simulink model "AUAV3_AND_SLUGS_SENSOR"  (Simulink 7.8)
settings: Solver=FixedStepDiscrete  StartTime=0.0  StopTime=10.0  FixedStep=T  RelTol=1e-3
PreLoadFcn:
  | T = 0.0025;
  | MavlinkBus;
  | 
  | % Baro Altitude Computation
  | % =========================
  | basePressure = 98192.64;
  | baseTemp = 288.215;
  | lapseRate = -0.00198122;
  | baseHeight = 0;
  | 
  | mcuInit
values from neighbouring files (symbols this model uses):
  apSampleTime = 0.01    [mcuInit.m]
  mavlink_gps_raw_int_t = Simulink.Bus    [MavlinkBus.m]    (also in MavlinkBusMarcello.m)
  mavlink_raw_imu_t = Simulink.Bus    [MavlinkBus.m]    (also in MavlinkBusMarcello.m)
  mavlink_scaled_pressure_t = Simulink.Bus    [MavlinkBus.m]    (also in MavlinkBusMarcello.m)
  mavlink_sys_status_t = Simulink.Bus    [MavlinkBus.m]    (also in MavlinkBusMarcello.m)
undefined symbols (not defined in the file or in its folder): A0, A14, A15, A2, A3, A5, A6, B0, barAdjust, baroCutTemp, baroOffset, baroScale, barTGain1, barTGain2, barTMean1, barTMean2, cubeAccelGain16405, cubeGyroGain16405, cubeMagGain16405, D0, D11, D8, G0, G15, gaind, IC1max, lowRateSensorCutoff, mainSensorCutoff, Max, maxDynPressure, ms, OC1max, P112, P127, P16, P21, P30, P31, P64, P72, P75, P80, P82, P83, Pin, pitAdjust, pitCutTemp, pitotOffset, pitotScale, pitTGain1, pitTGain2, pitTMean1, pitTMean2, polesd, powerOffset, powerScale, pressureSensorCutoff, Resol, tempOffset, tempScale ... (+5)
libraries: MCHP_Blockset x56, simulink x21, aerolibconvert2 x2
(part 3 of 5)

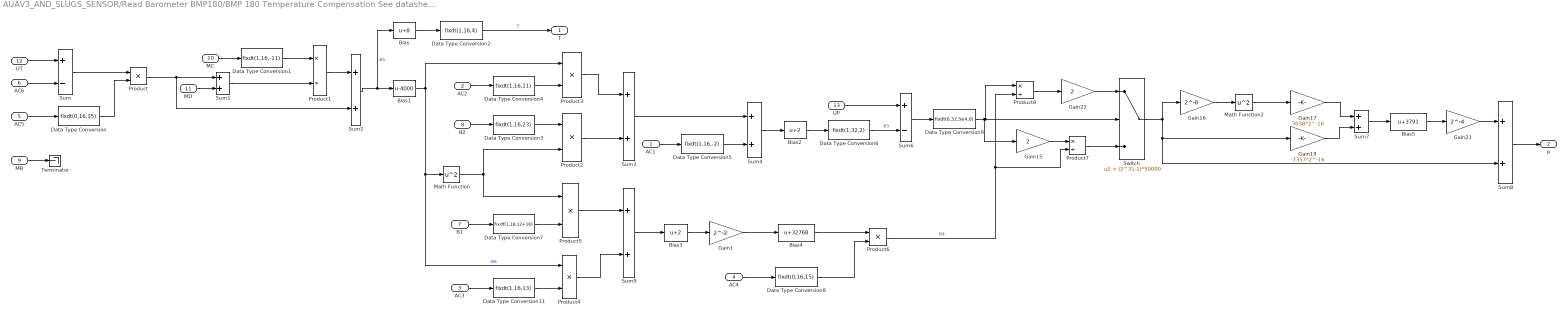
== system AUAV3_AND_SLUGS_SENSOR/Read Barometer BMP180/BMP 180 Temperature Compensation See datasheet ==
  AC1 : Inport
  AC2 : Inport  Port=2
  AC3 : Inport  Port=3
  AC4 : Inport  Port=4
  AC5 : Inport  Port=5
  AC6 : Inport  Port=6
  B1 : Inport  Port=7
  B2 : Inport  Port=8
  MB : Inport  Port=9
  MC : Inport  Port=10
  MD : Inport  Port=11
  UT : Inport  Port=12
  UP : Inport  Port=13
  Bias : Bias  Bias=8
  Bias1 : Bias  Bias=-4000
  Bias2 : Bias  Bias=2
  Bias3 : Bias  Bias=2
  Bias4 : Bias  Bias=32768
  Bias5 : Bias  Bias=3791
  Data Type Conversion : DataTypeConversion  OutDataTypeStr=fixdt(0,16,15)  ConvertRealWorld=Stored Integer (SI)
  Data Type Conversion1 : DataTypeConversion  OutDataTypeStr=fixdt(1,16,-11)  ConvertRealWorld=Stored Integer (SI)
  Data Type Conversion11 : DataTypeConversion  OutDataTypeStr=fixdt(1,16,13)  ConvertRealWorld=Stored Integer (SI)
  Data Type Conversion2 : DataTypeConversion  OutDataTypeStr=fixdt(1,16,4)  ConvertRealWorld=Stored Integer (SI)
  Data Type Conversion3 : DataTypeConversion  OutDataTypeStr=fixdt(1,16,23)  ConvertRealWorld=Stored Integer (SI)
  Data Type Conversion4 : DataTypeConversion  OutDataTypeStr=fixdt(1,16,11)  ConvertRealWorld=Stored Integer (SI)
  Data Type Conversion5 : DataTypeConversion  OutDataTypeStr=fixdt(1,16,-2)  ConvertRealWorld=Stored Integer (SI)
  Data Type Conversion6 : DataTypeConversion  OutDataTypeStr=fixdt(1,32,2)  ConvertRealWorld=Stored Integer (SI)
  Data Type Conversion7 : DataTypeConversion  OutDataTypeStr=fixdt(1,16,12+16)  ConvertRealWorld=Stored Integer (SI)
  Data Type Conversion8 : DataTypeConversion  OutDataTypeStr=fixdt(0,16,15)  ConvertRealWorld=Stored Integer (SI)
  Data Type Conversion9 : DataTypeConversion  OutDataTypeStr=fixdt(0,32,5e4,0)  ConvertRealWorld=Stored Integer (SI)
  Gain1 : Gain  Gain=2^-2  OutDataTypeStr=int32
  Gain15 : Gain  Gain=2  OutDataTypeStr=uint32  RndMeth=Round
  Gain16 : Gain  Gain=2^-8  OutDataTypeStr=int32  RndMeth=Round
  Gain17 : Gain  Gain=3038*2^-16  OutDataTypeStr=uint32
  Gain19 : Gain  Gain=-7357*2^-16  ParamDataTypeStr=fixdt(1,16)  OutDataTypeStr=int32
  Gain21 : Gain  Gain=2^-4  OutDataTypeStr=Inherit: Same as input
  Gain22 : Gain  Gain=2  OutDataTypeStr=Inherit: Same as input
  Math Function : Math  Operator=square  SaturateOnIntegerOverflow=on  OutDataTypeStr=Inherit: Inherit via internal rule
  Math Function2 : Math  Operator=square  OutDataTypeStr=uint32  SaturateOnIntegerOverflow=on
  Product : Product  RndMeth=Round  OutDataTypeStr=Inherit: Same as first input
  Product1 : Product  Inputs=*/  OutDataTypeStr=int16  RndMeth=Round
  Product2 : Product  OutDataTypeStr=int16
  Product3 : Product  OutDataTypeStr=Inherit: Same as first input
  Product4 : Product  OutDataTypeStr=int16
  Product5 : Product  OutDataTypeStr=int16
  Product6 : Product  OutDataTypeStr=uint32
  Product7 : Product  Inputs=*/  RndMeth=Round
  Product8 : Product  Inputs=*/  OutDataTypeStr=uint32  RndMeth=Round
  Sum : Sum  Inputs=+-  RndMeth=Round
  Sum1 : Sum  RndMeth=Round  OutDataTypeStr=Inherit: Same as first input
  Sum2 : Sum  AccumDataTypeStr=int16  OutDataTypeStr=int16  RndMeth=Round
  Sum3 : Sum
  Sum4 : Sum  OutDataTypeStr=int32
  Sum6 : Sum  Inputs=+-  AccumDataTypeStr=uint32  OutDataTypeStr=uint32
  Sum7 : Sum  AccumDataTypeStr=int32  OutDataTypeStr=int32
  Sum8 : Sum  AccumDataTypeStr=int32  OutDataTypeStr=Inherit: Same as accumulator  RndMeth=Round
  Sum9 : Sum
  Switch : Switch  Criteria=u2 > Threshold  Threshold=(2^31-1)*50000
  Terminator : Terminator
  T : Outport
  p : Outport  Port=2
  wires:
  MB/1 -> Terminator/1
  Sum9/1 -> Bias3/1
  Product4/1 -> Sum9/2
  Product5/1 -> Sum9/1
  Product2/1 -> Sum3/2
  Product3/1 -> Sum3/1
  Data Type Conversion3/1 -> Product2/1
  Data Type Conversion11/1 -> Product4/2
  Product1/1 -> Sum2/1
  Data Type Conversion8/1 -> Product6/2
  Data Type Conversion7/1 -> Product5/2
  Data Type Conversion4/1 -> Product3/2
  Math Function/1 -> Product5/1, Product2/2
  Data Type Conversion/1 -> Product/2
  Bias5/1 -> Gain21/1
  Sum8/1 -> p/1
  Gain21/1 -> Sum8/1
  Sum7/1 -> Bias5/1
  Gain17/1 -> Sum7/1
  Gain19/1 -> Sum7/2
  Math Function2/1 -> Gain17/1
  Gain16/1 -> Math Function2/1
  Switch/1 -> Gain19/1, Sum8/2, Gain16/1
  Product7/1 -> Switch/3
  Product8/1 -> Gain22/1
  Data Type Conversion9/1 -> Gain15/1, Product8/1, Switch/2
  Sum6/1 -> Data Type Conversion9/1
  UP/1 -> Sum6/1
  Data Type Conversion6/1 -> Sum6/2  "B3"
  Product6/1 -> Product8/2, Product7/2  "B4"
  Bias4/1 -> Product6/1
  AC4/1 -> Data Type Conversion8/1
  Gain1/1 -> Bias4/1
  Bias3/1 -> Gain1/1
  B1/1 -> Data Type Conversion7/1
  AC3/1 -> Data Type Conversion11/1
  Sum4/1 -> Bias2/1
  Data Type Conversion5/1 -> Sum4/2
  Bias2/1 -> Data Type Conversion6/1
  AC1/1 -> Data Type Conversion5/1
  Sum3/1 -> Sum4/1
  AC2/1 -> Data Type Conversion4/1
  B2/1 -> Data Type Conversion3/1
  Bias1/1 -> Product3/1, Product4/1, Math Function/1  "B6"
  MC/1 -> Data Type Conversion1/1
  Data Type Conversion2/1 -> T/1  "T"
  Bias/1 -> Data Type Conversion2/1
  Sum1/1 -> Product1/2
  Sum2/1 -> Bias1/1, Bias/1  "B5"
  Product/1 -> Sum1/1, Sum2/2
  MD/1 -> Sum1/2
  AC5/1 -> Data Type Conversion/1
  Sum/1 -> Product/1
  AC6/1 -> Sum/2
  UT/1 -> Sum/1
  Data Type Conversion1/1 -> Product1/1
  Gain22/1 -> Switch/1
  Gain15/1 -> Product7/1

== system AUAV3_AND_SLUGS_SENSOR/Read Barometer BMP180/Baro Altimeter ==
  Static (Pa) : Inport
  Compute Barometric Height : Subsystem  mask{baseTemp=baseTemp, LapseRate=lapseRate}
      mask prompts: baseTemp "Base Station Temperature (K)"; LapseRate "Lapse Rate (C/ft)"
      mask help:
      | Produces Altitude in meters from Barometric Pressure in Pascals. Altitude is valid from MSL to 6000 ft.
      |
      | The method implemented here was developed by Ren Curry
  Constant5 : Constant  Value=baseHeight  OutDataTypeStr=single
  Enabled Subsystem : Subsystem  TreatAsAtomicUnit=on
  Enables/Disables the Computation of  initial Baro Bias : MATLAB Function  TreatAsAtomicUnit=on
  Initial Baro Bias : Subsystem  TreatAsAtomicUnit=on
  Logical Operator : Logic  Operator=NOT  AllPortsSameDT=off  OutDataTypeStr=boolean
  Sum1 : Sum  Inputs=++|  OutDataTypeStr=single
  Zero Out Height : Subsystem  TreatAsAtomicUnit=on
  Altitude : Outport
  wires:
  Enabled Subsystem/1(Out1) -> Altitude/1
  Sum1/1 -> Enabled Subsystem/1(In1)
  Logical Operator/1 -> Enabled Subsystem/Enable
  Zero Out Height/1(Height Offset) -> Sum1/1
  Initial Baro Bias/1(Baro (Gnd)) -> Compute Barometric Height/2(Base Pressure (Pa))
  Constant5/1 -> Zero Out Height/1(Base Height), Compute Barometric Height/1(Base Height (m))
  Enables/Disables the Computation of  initial Baro Bias/1(tOut) -> Logical Operator/1, Zero Out Height/Enable, Initial Baro Bias/Enable
  Static (Pa)/1 -> Compute Barometric Height/3(Baro (Pa)), Initial Baro Bias/1(Baro (Pa))
  Compute Barometric Height/1("Altitude, m") -> Sum1/2, Zero Out Height/2(Computed Height)

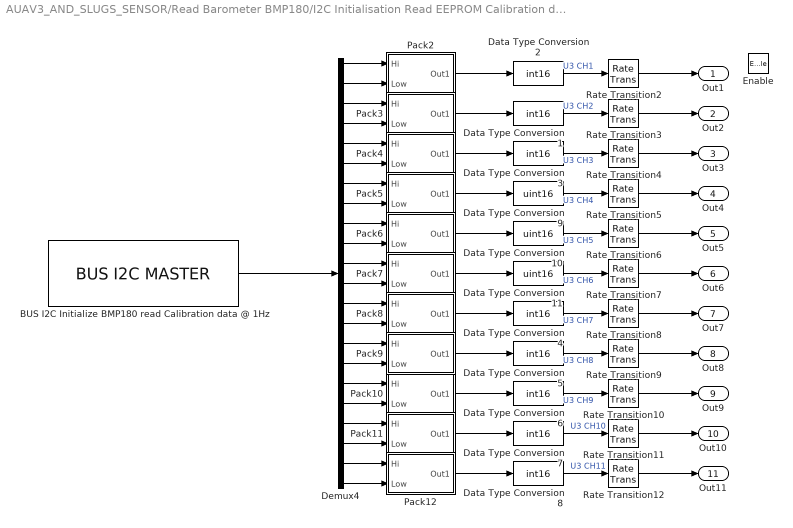
== system AUAV3_AND_SLUGS_SENSOR/Read Barometer BMP180/I2C Initialisation Read EEPROM Calibration data Once (Blocking Function) ==
  Enable : EnablePort
  BUS I2C Initialize BMP180 read Calibration data @ 1Hz : MCHP_Blockset/BUS I2C/BUS I2C MASTER  I2CRef=2  I2C_IntPriority=6  I2Csequence_txt="Initial-Configuration$     ---     $Start$Write Address:{[0x77]}    % BMP180 Address$Write Data (x1)  Write:{[0xAA ]}  $Re-Start    % Re-Start when not followed with either Read or Write action rethrow Address$Read Data (x22)  Read:{Out 9}$Stop"  I2Csequence_num=[BFF0000000000000 40E0600000000000 41186A0000000000 4118666E3C87173F]$[4070000000000000]$[3FF0000000000000 40E0200000000000 40F86A0000000000 40F866E066594CA2]$[4040000000000000 0000000000000000 0000000000000000 405DC00000000000]$[4050000000000000 3FF0000000000000 0000000000000000 4065400000000000]$[4008000000000000 40E0000000000000 40F86A0000000000 410065D9C7810E65]$[4060000000000000 4036000000000000]$[4000000000000000 40E0600000000000 40F86A0000000000 410065D9C7810E65]  InitialConfigurationNum=0  PIN_SDA_TXT=A3 / Pin[59]  PIN_SCL_TXT=A2 / Pin[58]  S_INPUT="[5  5]"  S_OUTPUT=[5]  S_INPUT_Size="[2  2]"  S_OUTPUT_Size=[4]  BlockingMode=on  SampleTime=.01  MCHP_MASTERLINK=|  MCHP_PORT={I2C 2 Clock}{SCL2}13:0:A2;{I2C 2 SDA}{SDA2}13:0:A3;  ORDERING=0
      | AUAV3_AND_SLUGS_SENSOR/Microchip Master
      | AUAV V3 Board
      | Busy Flag on D2 (RA6)
  Data Type Conversion{1..8} (8 alike) : DataTypeConversion  OutDataTypeStr=int16  ConvertRealWorld=Stored Integer (SI)
  Data Type Conversion10 : DataTypeConversion  OutDataTypeStr=uint16  ConvertRealWorld=Stored Integer (SI)  LockScale=on
  Data Type Conversion11 : DataTypeConversion  OutDataTypeStr=uint16  ConvertRealWorld=Stored Integer (SI)  LockScale=on
  Data Type Conversion9 : DataTypeConversion  OutDataTypeStr=uint16  ConvertRealWorld=Stored Integer (SI)  LockScale=on
  Demux4 : Demux  Outputs=22
  Pack10 : Subsystem
  Pack11 : Subsystem
  Pack12 : Subsystem
  Pack2 : Subsystem
  Pack3 : Subsystem
  Pack4 : Subsystem
  Pack5 : Subsystem
  Pack6 : Subsystem
  Pack7 : Subsystem
  Pack8 : Subsystem
  Pack9 : Subsystem
  Rate Transition{2..12} (11 alike) : RateTransition  Deterministic=off
  Out1 : Outport
  Out2 : Outport  Port=2
  Out3 : Outport  Port=3
  Out4 : Outport  Port=4
  Out5 : Outport  Port=5
  Out6 : Outport  Port=6
  Out7 : Outport  Port=7
  Out8 : Outport  Port=8
  Out9 : Outport  Port=9
  Out10 : Outport  Port=10
  Out11 : Outport  Port=11
  wires:
  BUS I2C Initialize BMP180 read Calibration data @ 1Hz/1 -> Demux4/1
  Demux4/12 -> Pack7/2(Low)
  Data Type Conversion10/1 -> Rate Transition6/1  "U3 CH5"
  Data Type Conversion1/1 -> Rate Transition3/1  "U3 CH2"
  Data Type Conversion2/1 -> Rate Transition2/1  "U3 CH1"
  Data Type Conversion11/1 -> Rate Transition7/1  "U3 CH6"
  Data Type Conversion5/1 -> Rate Transition9/1  "U3 CH8"
  Data Type Conversion8/1 -> Rate Transition12/1  "U3 CH11"
  Data Type Conversion6/1 -> Rate Transition10/1  "U3 CH9"
  Data Type Conversion4/1 -> Rate Transition8/1  "U3 CH7"
  Data Type Conversion3/1 -> Rate Transition4/1  "U3 CH3"
  Data Type Conversion7/1 -> Rate Transition11/1  "U3 CH10"
  Data Type Conversion9/1 -> Rate Transition5/1  "U3 CH4"
  Pack6/1(Out1) -> Data Type Conversion10/1
  Pack5/1(Out1) -> Data Type Conversion9/1
  Pack7/1(Out1) -> Data Type Conversion11/1
  Pack8/1(Out1) -> Data Type Conversion4/1
  Pack9/1(Out1) -> Data Type Conversion5/1
  Pack10/1(Out1) -> Data Type Conversion6/1
  Pack11/1(Out1) -> Data Type Conversion7/1
  Pack12/1(Out1) -> Data Type Conversion8/1
  Pack4/1(Out1) -> Data Type Conversion3/1
  Demux4/15 -> Pack9/1(Hi)
  Pack3/1(Out1) -> Data Type Conversion1/1
  Pack2/1(Out1) -> Data Type Conversion2/1
  Demux4/22 -> Pack12/2(Low)
  Demux4/14 -> Pack8/2(Low)
  Demux4/16 -> Pack9/2(Low)
  Demux4/17 -> Pack10/1(Hi)
  Demux4/18 -> Pack10/2(Low)
  Demux4/19 -> Pack11/1(Hi)
  Demux4/20 -> Pack11/2(Low)
  Demux4/21 -> Pack12/1(Hi)
  Demux4/2 -> Pack2/2(Low)
  Demux4/13 -> Pack8/1(Hi)
  Demux4/11 -> Pack7/1(Hi)
  Demux4/9 -> Pack6/1(Hi)
  Demux4/10 -> Pack6/2(Low)
  Demux4/1 -> Pack2/1(Hi)
  Demux4/3 -> Pack3/1(Hi)
  Demux4/4 -> Pack3/2(Low)
  Demux4/6 -> Pack4/2(Low)
  Demux4/5 -> Pack4/1(Hi)
  Demux4/7 -> Pack5/1(Hi)
  Demux4/8 -> Pack5/2(Low)
  Rate Transition12/1 -> Out11/1
  Rate Transition10/1 -> Out9/1
  Rate Transition11/1 -> Out10/1
  Rate Transition9/1 -> Out8/1
  Rate Transition3/1 -> Out2/1
  Rate Transition7/1 -> Out6/1
  Rate Transition4/1 -> Out3/1
  Rate Transition6/1 -> Out5/1
  Rate Transition8/1 -> Out7/1
  Rate Transition2/1 -> Out1/1
  Rate Transition5/1 -> Out4/1

== system AUAV3_AND_SLUGS_SENSOR/Read Barometer BMP180/LPF 1Hz ==
  Input : Inport
  Delay11 : Delay  DelayLength=1  InitialCondition=0  InputProcessing=Inherited
  SumA21 : Sum  Inputs=|++  AccumDataTypeStr=fixdt(0,32,15)  OutDataTypeStr=Inherit: Same as accumulator  SaturateOnIntegerOverflow=on
  SumB21 : Sum  Inputs=|++  AccumDataTypeStr=fixdt(0,32,16)  OutDataTypeStr=uint16  SaturateOnIntegerOverflow=on
  a(2)(1) : Gain  Gain=0.9390625058174924  ParamDataTypeStr=fixdt(0,16,16)  OutDataTypeStr=fixdt(0,32,15)  SaturateOnIntegerOverflow=on
  s(1) : Gain  Gain=0.030468747091253828  ParamDataTypeStr=fixdt(0,16,20)  OutDataTypeStr=fixdt(0,32,16)  SaturateOnIntegerOverflow=on
  Output : Outport
  wires:
  s(1)/1 -> SumA21/1
  SumA21/1 -> SumB21/1, Delay11/1
  a(2)(1)/1 -> SumA21/2
  Delay11/1 -> SumB21/2, a(2)(1)/1
  SumB21/1 -> Output/1
  Input/1 -> s(1)/1

== system AUAV3_AND_SLUGS_SENSOR/Read Barometer BMP180/LPF 1Hz1 ==
  Input : Inport
  Delay11 : Delay  DelayLength=1  InitialCondition=0  InputProcessing=Inherited
  SumA21 : Sum  Inputs=|++  AccumDataTypeStr=fixdt(0,32,15)  OutDataTypeStr=Inherit: Same as accumulator  SaturateOnIntegerOverflow=on
  SumB21 : Sum  Inputs=|++  AccumDataTypeStr=fixdt(0,32,16)  OutDataTypeStr=uint16  SaturateOnIntegerOverflow=on
  a(2)(1) : Gain  Gain=0.9390625058174924  ParamDataTypeStr=fixdt(0,16,16)  OutDataTypeStr=fixdt(0,32,15)  SaturateOnIntegerOverflow=on
  s(1) : Gain  Gain=0.030468747091253828  ParamDataTypeStr=fixdt(0,16,20)  OutDataTypeStr=fixdt(0,32,16)  SaturateOnIntegerOverflow=on
  Output : Outport
  wires:
  Input/1 -> s(1)/1
  SumB21/1 -> Output/1
  Delay11/1 -> a(2)(1)/1, SumB21/2
  a(2)(1)/1 -> SumA21/2
  SumA21/1 -> Delay11/1, SumB21/1
  s(1)/1 -> SumA21/1

== system AUAV3_AND_SLUGS_SENSOR/Read Barometer BMP180/Pack ==
  Hi : Inport
  Low : Inport  Port=2
  Bitwise Operator : simulink/Logic and Bit Operations/Bitwise Operator  logicop=OR  UseBitMask=off  NumInputPorts=2  BitMask=bin2dec('11011001')  BitMaskRealWorld=Stored Integer
  Data Type Conversion1 : DataTypeConversion  OutDataTypeStr=uint16  ConvertRealWorld=Stored Integer (SI)
  Data Type Conversion2 : DataTypeConversion  OutDataTypeStr=uint16  ConvertRealWorld=Stored Integer (SI)
  Data Type Conversion3 : DataTypeConversion  OutDataTypeStr=uint16  ConvertRealWorld=Stored Integer (SI)
  Gain : Gain  Gain=2^8  OutDataTypeStr=Inherit: Same as input
  Out1 : Outport
  wires:
  Data Type Conversion3/1 -> Bitwise Operator/2
  Low/1 -> Data Type Conversion3/1
  Data Type Conversion1/1 -> Gain/1
  Bitwise Operator/1 -> Data Type Conversion2/1
  Hi/1 -> Data Type Conversion1/1
  Gain/1 -> Bitwise Operator/1
  Data Type Conversion2/1 -> Out1/1

== system AUAV3_AND_SLUGS_SENSOR/Read Barometer BMP180/Pack1 ==
  Hi : Inport
  Low : Inport  Port=2
  Bitwise Operator : simulink/Logic and Bit Operations/Bitwise Operator  logicop=OR  UseBitMask=off  NumInputPorts=2  BitMask=bin2dec('11011001')  BitMaskRealWorld=Stored Integer
  Data Type Conversion1 : DataTypeConversion  OutDataTypeStr=uint16  ConvertRealWorld=Stored Integer (SI)
  Data Type Conversion2 : DataTypeConversion  OutDataTypeStr=uint16  ConvertRealWorld=Stored Integer (SI)
  Data Type Conversion3 : DataTypeConversion  OutDataTypeStr=uint16  ConvertRealWorld=Stored Integer (SI)
  Gain : Gain  Gain=2^8  OutDataTypeStr=Inherit: Same as input
  Out1 : Outport
  wires:
  Gain/1 -> Bitwise Operator/1
  Hi/1 -> Data Type Conversion1/1
  Bitwise Operator/1 -> Data Type Conversion2/1
  Data Type Conversion1/1 -> Gain/1
  Low/1 -> Data Type Conversion3/1
  Data Type Conversion3/1 -> Bitwise Operator/2
  Data Type Conversion2/1 -> Out1/1

== system AUAV3_AND_SLUGS_SENSOR/Read MPU600 and HMC5883/Subsystem10 ==
  Hi : Inport
  Low : Inport  Port=2
  Bitwise Operator : simulink/Logic and Bit Operations/Bitwise Operator  logicop=OR  UseBitMask=off  NumInputPorts=2  BitMask=bin2dec('11011001')  BitMaskRealWorld=Stored Integer
  Data Type Conversion1 : DataTypeConversion  OutDataTypeStr=uint16  ConvertRealWorld=Stored Integer (SI)
  Data Type Conversion2 : DataTypeConversion  OutDataTypeStr=int16  ConvertRealWorld=Stored Integer (SI)
  Data Type Conversion3 : DataTypeConversion  OutDataTypeStr=uint16  ConvertRealWorld=Stored Integer (SI)
  Shift Arithmetic : ArithShift  BitShiftNumber=8
  Out1 : Outport
  wires:
  Hi/1 -> Data Type Conversion1/1
  Bitwise Operator/1 -> Data Type Conversion2/1
  Data Type Conversion2/1 -> Out1/1
  Data Type Conversion1/1 -> Shift Arithmetic/1
  Shift Arithmetic/1 -> Bitwise Operator/1
  Low/1 -> Data Type Conversion3/1
  Data Type Conversion3/1 -> Bitwise Operator/2

== system AUAV3_AND_SLUGS_SENSOR/Read MPU600 and HMC5883/Subsystem8 ==
  Hi : Inport
  Low : Inport  Port=2
  Bitwise Operator : simulink/Logic and Bit Operations/Bitwise Operator  logicop=OR  UseBitMask=off  NumInputPorts=2  BitMask=bin2dec('11011001')  BitMaskRealWorld=Stored Integer
  Data Type Conversion1 : DataTypeConversion  OutDataTypeStr=uint16  ConvertRealWorld=Stored Integer (SI)
  Data Type Conversion2 : DataTypeConversion  OutDataTypeStr=int16  ConvertRealWorld=Stored Integer (SI)
  Data Type Conversion3 : DataTypeConversion  OutDataTypeStr=uint16  ConvertRealWorld=Stored Integer (SI)
  Shift Arithmetic : ArithShift  BitShiftNumber=8
  Out1 : Outport
  wires:
  Hi/1 -> Data Type Conversion1/1
  Bitwise Operator/1 -> Data Type Conversion2/1
  Data Type Conversion2/1 -> Out1/1
  Data Type Conversion1/1 -> Shift Arithmetic/1
  Shift Arithmetic/1 -> Bitwise Operator/1
  Low/1 -> Data Type Conversion3/1
  Data Type Conversion3/1 -> Bitwise Operator/2

== system AUAV3_AND_SLUGS_SENSOR/Read MPU600 and HMC5883/Subsystem9 ==
  Hi : Inport
  Low : Inport  Port=2
  Bitwise Operator : simulink/Logic and Bit Operations/Bitwise Operator  logicop=OR  UseBitMask=off  NumInputPorts=2  BitMask=bin2dec('11011001')  BitMaskRealWorld=Stored Integer
  Data Type Conversion1 : DataTypeConversion  OutDataTypeStr=uint16  ConvertRealWorld=Stored Integer (SI)
  Data Type Conversion2 : DataTypeConversion  OutDataTypeStr=int16  ConvertRealWorld=Stored Integer (SI)
  Data Type Conversion3 : DataTypeConversion  OutDataTypeStr=uint16  ConvertRealWorld=Stored Integer (SI)
  Shift Arithmetic : ArithShift  BitShiftNumber=8
  Out1 : Outport
  wires:
  Data Type Conversion3/1 -> Bitwise Operator/2
  Low/1 -> Data Type Conversion3/1
  Shift Arithmetic/1 -> Bitwise Operator/1
  Data Type Conversion1/1 -> Shift Arithmetic/1
  Data Type Conversion2/1 -> Out1/1
  Bitwise Operator/1 -> Data Type Conversion2/1
  Hi/1 -> Data Type Conversion1/1

== system AUAV3_AND_SLUGS_SENSOR/Sensor Data/Raw HIL  Readings ==
  Enable : EnablePort
  Data from HIL [hil.c]2 : MCHP_Blockset/User Functions/C Function Call  ParseFilesChkbx=off  ListFunctions1=Custom Function  Function1=extern void hilRead(uint8_T* y1);  AddHeaderDeclaration=off  Function1Type=when block is updated (default)  FctReturnBlockOut=on  Fct1BlockOut=y1[13]  DataCollected=0  ORDERING=None  SampleTime=.01  MCHP_MASTERLINK=|  PinDigitalInput=[]  PinDigitalOutput=[]  PinAnalogInput=[]
      | AUAV3_AND_SLUGS_SENSOR/Microchip Master
      | AUAV V3 Board
      | Busy Flag on D2 (RA6)
  HIL Messages  Parser/Decoder [hil.c]1 : MCHP_Blockset/User Functions/C Function Call  ParseFilesChkbx=off  ListFunctions1=Custom Function  Function1=extern void protDecodeHil(uint8_T* u1);  AddHeaderDeclaration=off  Function1Type=when block is updated (default)  Fct1BlockIn=u1[13]  FctReturnBlockOut=off  Fct1BlockOut=u1[13]  DataCollected=0  ORDERING=None  SampleTime=-1  MCHP_MASTERLINK=|  PinDigitalInput=[]  PinDigitalOutput=[]  PinAnalogInput=[]
      | AUAV3_AND_SLUGS_SENSOR/Microchip Master
      | AUAV V3 Board
      | Busy Flag on D2 (RA6)
  HIL Raw Readings [hil.c]1 : MCHP_Blockset/User Functions/C Function Call  ParseFilesChkbx=off  ListFunctions1=Custom Function  Function1=extern void hil_getRawRead(uint8_T* y1);  AddHeaderDeclaration=off  Function1Type=when block is updated (default)  Fct1BlockIn=y1[13]  FctReturnBlockOut=off  Fct1BlockOut=y1[13]  ORDERING=None  SampleTime=-1  MCHP_MASTERLINK=|  PinDigitalInput=[]  PinDigitalOutput=[]  PinAnalogInput=[]
      | AUAV3_AND_SLUGS_SENSOR/Microchip Master
      | AUAV V3 Board
      | Busy Flag on D2 (RA6)
  Raw Msg : Outport
  wires:
  Data from HIL [hil.c]2/1 -> HIL Messages  Parser/Decoder [hil.c]1/1
  HIL Messages  Parser/Decoder [hil.c]1/1 -> HIL Raw Readings [hil.c]1/1
  HIL Raw Readings [hil.c]1/1 -> Raw Msg/1

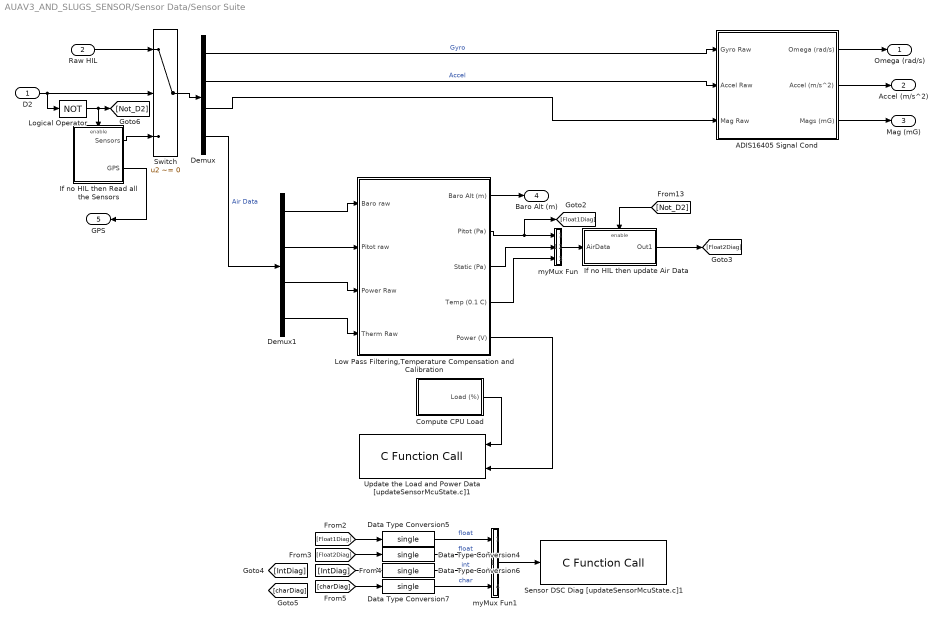
== system AUAV3_AND_SLUGS_SENSOR/Sensor Data/Sensor Suite ==
  D2 : Inport
  Raw HIL : Inport  Port=2
  "ADIS16405 Signal Cond " : Subsystem
  Compute CPU Load : Subsystem
  Data Type Conversion{4..7} (4 alike) : DataTypeConversion  OutDataTypeStr=single
  Demux : Demux  Outputs=[3 3 3 4]
  Demux1 : Demux
  If no HIL then Read all the Sensors : Subsystem
  If no HIL then update Air Data : Subsystem
  Logical Operator : Logic  Operator=NOT  AllPortsSameDT=off  OutDataTypeStr=boolean
  Low Pass Filtering,Temperature Compensation and Calibration : Subsystem
  Sensor DSC Diag [updateSensorMcuState.c]1 : MCHP_Blockset/User Functions/C Function Call  ParseFilesChkbx=off  ListFunctions1=Custom Function  Function1=extern void updateSensorDiag(real32_T* u1);  AddHeaderDeclaration=off  Function1Type=when block is updated (default)  Fct1BlockIn=u1[4]  FctReturnBlockOut=off  DataCollected=0  ORDERING=None  SampleTime=.01  MCHP_MASTERLINK=|  PinDigitalInput=[]  PinDigitalOutput=[]  PinAnalogInput=[]
      | AUAV3_AND_SLUGS_SENSOR/Microchip Master
      | AUAV V3 Board
      | Busy Flag on D2 (RA6)
  Switch : Switch  Criteria=u2 ~= 0  SampleTime=0.01
  Update the Load and Power Data [updateSensorMcuState.c]1 : MCHP_Blockset/User Functions/C Function Call  ParseFilesChkbx=off  ListFunctions1=Custom Function  Function1=extern void updateLoadData(uint8_T u1, uint16_T u2);  AddHeaderDeclaration=off  Function1Type=when block is updated (default)  FctReturnBlockOut=off  DataCollected=0  ORDERING=None  SampleTime=.01  MCHP_MASTERLINK=|  PinDigitalInput=[]  PinDigitalOutput=[]  PinAnalogInput=[]
      | AUAV3_AND_SLUGS_SENSOR/Microchip Master
      | AUAV V3 Board
      | Busy Flag on D2 (RA6)
  myMux Fun : MATLAB Function  TreatAsAtomicUnit=on
  myMux Fun1 : MATLAB Function  TreatAsAtomicUnit=on
  Omega (rad/s) : Outport
  Accel (m/s^2) : Outport  Port=2
  Mag (mG) : Outport  Port=3
  Baro Alt (m) : Outport  Port=4
  GPS : Outport  Port=5
  wires:
  Switch/1 -> Demux/1
  D2/1 -> Switch/2, Logical Operator/1
  If no HIL then Read all the Sensors/1(Sensors) -> Switch/3
  Logical Operator/1 -> If no HIL then Read all the Sensors/Enable, [Not_D2]
  Raw HIL/1 -> Switch/1
  Low Pass Filtering,Temperature Compensation and Calibration/1(Baro Alt (m)) -> Baro Alt (m)/1
  Demux/1 -> "ADIS16405 Signal Cond "/1(Gyro Raw)  "Gyro"
  Demux/4 -> Demux1/1  "Air Data"
  Demux1/1 -> Low Pass Filtering,Temperature Compensation and Calibration/1(Baro raw)
  Demux1/2 -> Low Pass Filtering,Temperature Compensation and Calibration/2(Pitot raw)
  Demux1/4 -> Low Pass Filtering,Temperature Compensation and Calibration/4(Therm Raw)
  Demux/3 -> "ADIS16405 Signal Cond "/3(Mag Raw)
  Demux1/3 -> Low Pass Filtering,Temperature Compensation and Calibration/3(Power Raw)
  Low Pass Filtering,Temperature Compensation and Calibration/2(Pitot (Pa)) -> myMux Fun/1(u1), [Float1Diag]
  Low Pass Filtering,Temperature Compensation and Calibration/3(Static (Pa)) -> myMux Fun/2(u2)
  myMux Fun/1(y) -> If no HIL then update Air Data/1(AirData)
  Low Pass Filtering,Temperature Compensation and Calibration/4(Temp (0.1 C)) -> myMux Fun/3(u3)
  Compute CPU Load/1(Load (%)) -> Update the Load and Power Data [updateSensorMcuState.c]1/1
  Low Pass Filtering,Temperature Compensation and Calibration/5(Power (V)) -> Update the Load and Power Data [updateSensorMcuState.c]1/2
  If no HIL then Read all the Sensors/2(GPS) -> GPS/1
  Demux/2 -> "ADIS16405 Signal Cond "/2(Accel Raw)  "Accel"
  myMux Fun1/1(y) -> Sensor DSC Diag [updateSensorMcuState.c]1/1
  Data Type Conversion5/1 -> myMux Fun1/1(u1)  "float"
  Data Type Conversion4/1 -> myMux Fun1/2(u2)  "float"
  Data Type Conversion6/1 -> myMux Fun1/3(u3)  "int"
  Data Type Conversion7/1 -> myMux Fun1/4(u4)  "char"
  [Float1Diag] -> Data Type Conversion5/1
  [Float2Diag] -> Data Type Conversion4/1
  [IntDiag] -> Data Type Conversion6/1
  [charDiag] -> Data Type Conversion7/1
  "ADIS16405 Signal Cond "/1(Omega (rad/s)) -> Omega (rad/s)/1
  "ADIS16405 Signal Cond "/2(Accel (m/s^2)) -> Accel (m/s^2)/1
  "ADIS16405 Signal Cond "/3(Mags (mG)) -> Mag (mG)/1
  [Not_D2] -> If no HIL then update Air Data/Enable
  If no HIL then update Air Data/1(Out1) -> [Float2Diag]

== system AUAV3_AND_SLUGS_SENSOR/Servo In Out/Mixing ==
  note: Pitch positif : go down
      | Yaw positive : turn left
  Pitch : Inport
  Roll : Inport  Port=2
  Sum : Sum  Inputs=-+  SaturateOnIntegerOverflow=on  OutDataTypeStr=Inherit: Same as first input
  Sum1 : Sum  SaturateOnIntegerOverflow=on  OutDataTypeStr=Inherit: Same as first input
  Cmd Servo Left : Outport
  Cmd Servo Right : Outport  Port=2
  wires:
  Pitch/1 -> Sum1/1, Sum/1
  Roll/1 -> Sum/2, Sum1/2
  Sum/1 -> Cmd Servo Left/1
  Sum1/1 -> Cmd Servo Right/1

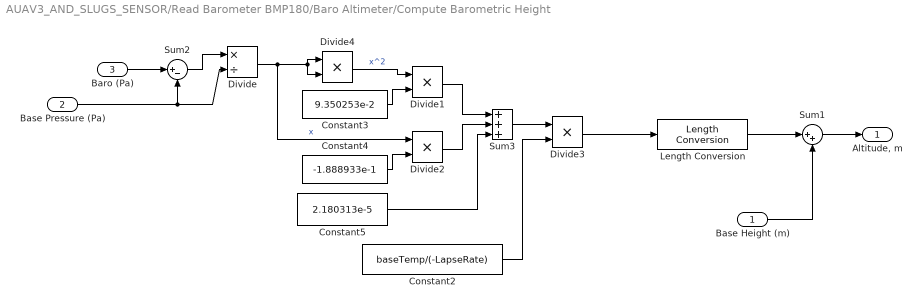
== system AUAV3_AND_SLUGS_SENSOR/Read Barometer BMP180/Baro Altimeter/Compute Barometric Height ==
  Base Height (m) : Inport
  Base Pressure (Pa) : Inport  Port=2
  Baro (Pa) : Inport  Port=3
  Constant2 : Constant  Value=baseTemp/(-LapseRate)  OutDataTypeStr=single
  Constant3 : Constant  Value=9.350253e-2  OutDataTypeStr=single
  Constant4 : Constant  Value=-1.888933e-1  OutDataTypeStr=single
  Constant5 : Constant  Value=2.180313e-5  OutDataTypeStr=single
  Divide : Product  Inputs=*/  OutDataTypeStr=single
  Divide{1..4} (4 alike) : Product  OutDataTypeStr=single
  Length Conversion : aerolibconvert2/Length Conversion  IU=ft  OU=m
  Sum1 : Sum  Inputs=|++  OutDataTypeStr=single
  Sum2 : Sum  Inputs=|+-  OutDataTypeStr=single
  Sum3 : Sum  Inputs=3  OutDataTypeStr=single
  "Altitude, m" : Outport
  wires:
  Baro (Pa)/1 -> Sum2/1
  Base Height (m)/1 -> Sum1/2
  Base Pressure (Pa)/1 -> Sum2/2, Divide/2
  Divide/1 -> Divide4/2, Divide4/1, Divide2/1  "x"
  Divide4/1 -> Divide1/1  "x^2"
  Constant3/1 -> Divide1/2
  Constant4/1 -> Divide2/2
  Divide1/1 -> Sum3/1
  Divide2/1 -> Sum3/2
  Constant5/1 -> Sum3/3
  Sum3/1 -> Divide3/1
  Constant2/1 -> Divide3/2
  Divide3/1 -> Length Conversion/1
  Sum1/1 -> "Altitude, m"/1
  Sum2/1 -> Divide/1
  Length Conversion/1 -> Sum1/1

== system AUAV3_AND_SLUGS_SENSOR/Read Barometer BMP180/Baro Altimeter/Enabled Subsystem ==
  In1 : Inport
  Enable : EnablePort
  Out1 : Outport  InitialOutput=baseHeight
  wires:
  In1/1 -> Out1/1

== system AUAV3_AND_SLUGS_SENSOR/Read Barometer BMP180/Baro Altimeter/Initial Baro Bias ==
  Baro (Pa) : Inport
  Enable : EnablePort
  Data Type Conversion : DataTypeConversion  OutDataTypeStr=double
  Data Type Conversion1 : DataTypeConversion  OutDataTypeStr=single
  Low Pass8 : Subsystem  mask(DiscretizedZeroPole){Zeros=[], Poles=[-3], Gain=3, AbsTol=auto, SampleTime=.01, method=tustin, Wc=1}
      mask prompts: Zeros "Zeros (enter in s-main:)"; Poles "Poles (enter in s-domain:)"; Gain "Gain (enter in s-domain:)"; AbsTol "Absolute tolerance:"; SampleTime "Sample time:"; Wc "Critical Frequency (Hz):"
      mask help: Continuous mask uses c2d to transform parameters onto the Discrete Zero-Pole block inside.
      mask init:
      | st=SampleTime;
      | if length(st)>1
      |     st=SampleTime(1);
      | end
      | if(st>0)
      |     [zerosd,polesd,gaind] = sldiscutil('disczpk', {st,method,Wc,Zeros,Poles,Gain});
      | end	
      | s = get_param(gcb,'maskvalues');
      | zeross = s{1};
      | poless = s{2};
      | gainss = s{3};
      | %zerosc = eval(zeross);
      | %polesc = eval(poless);
      | %gainsc = eval(gainss);
      | sldiscutil('initzpkmask', st);
      | if(st==0)
      | set_param([gcb '/Zero Pole'], 'AbsoluteTolerance', AbsTol);
      | end
      mask StyleString: edit,edit,edit,edit,edit,popup(zoh|foh|tustin|prewarp|matched),edit
      mask CallbackString: |||||hidecrit|
      mask Display:
      | droots(zeross,poless,gainss)
      | text( 0.5, 1.0, method, 'verticalAlignment','top')
  "[80k - 120k]" : Saturate  UpperLimit=120000  LowerLimit=80000
  Baro (Gnd) : Outport
  wires:
  "[80k - 120k]"/1 -> Baro (Gnd)/1
  Data Type Conversion1/1 -> "[80k - 120k]"/1
  Data Type Conversion/1 -> Low Pass8/1(In1)
  Low Pass8/1(Out1) -> Data Type Conversion1/1
  Baro (Pa)/1 -> Data Type Conversion/1

== system AUAV3_AND_SLUGS_SENSOR/Read Barometer BMP180/Baro Altimeter/Zero Out Height ==
  Base Height : Inport
  Computed Height : Inport  Port=2
  Enable : EnablePort
  Integer Delay : Delay  DelayLength=1  InitialCondition=0  InputProcessing=Inherited  SampleTime=.01
  Sum : Sum  Inputs=|+-  OutDataTypeStr=single
  Height Offset : Outport
  wires:
  Base Height/1 -> Sum/1
  Integer Delay/1 -> Sum/2
  Sum/1 -> Height Offset/1
  Computed Height/1 -> Integer Delay/1

== system AUAV3_AND_SLUGS_SENSOR/Read Barometer BMP180/I2C Initialisation Read EEPROM Calibration data Once (Blocking Function)/Pack10 ==
  Hi : Inport
  Low : Inport  Port=2
  Bitwise Operator : simulink/Logic and Bit Operations/Bitwise Operator  logicop=OR  UseBitMask=off  NumInputPorts=2  BitMask=bin2dec('11011001')  BitMaskRealWorld=Stored Integer
  Data Type Conversion1 : DataTypeConversion  OutDataTypeStr=uint16  ConvertRealWorld=Stored Integer (SI)
  Data Type Conversion2 : DataTypeConversion  OutDataTypeStr=uint16  ConvertRealWorld=Stored Integer (SI)
  Data Type Conversion3 : DataTypeConversion  OutDataTypeStr=uint16  ConvertRealWorld=Stored Integer (SI)
  Gain : Gain  Gain=2^8  OutDataTypeStr=Inherit: Same as input
  Out1 : Outport
  wires:
  Data Type Conversion3/1 -> Bitwise Operator/2
  Low/1 -> Data Type Conversion3/1
  Data Type Conversion1/1 -> Gain/1
  Bitwise Operator/1 -> Data Type Conversion2/1
  Hi/1 -> Data Type Conversion1/1
  Gain/1 -> Bitwise Operator/1
  Data Type Conversion2/1 -> Out1/1

== system AUAV3_AND_SLUGS_SENSOR/Read Barometer BMP180/I2C Initialisation Read EEPROM Calibration data Once (Blocking Function)/Pack11 ==
  Hi : Inport
  Low : Inport  Port=2
  Bitwise Operator : simulink/Logic and Bit Operations/Bitwise Operator  logicop=OR  UseBitMask=off  NumInputPorts=2  BitMask=bin2dec('11011001')  BitMaskRealWorld=Stored Integer
  Data Type Conversion1 : DataTypeConversion  OutDataTypeStr=uint16  ConvertRealWorld=Stored Integer (SI)
  Data Type Conversion2 : DataTypeConversion  OutDataTypeStr=uint16  ConvertRealWorld=Stored Integer (SI)
  Data Type Conversion3 : DataTypeConversion  OutDataTypeStr=uint16  ConvertRealWorld=Stored Integer (SI)
  Gain : Gain  Gain=2^8  OutDataTypeStr=Inherit: Same as input
  Out1 : Outport
  wires:
  Data Type Conversion3/1 -> Bitwise Operator/2
  Low/1 -> Data Type Conversion3/1
  Data Type Conversion1/1 -> Gain/1
  Bitwise Operator/1 -> Data Type Conversion2/1
  Hi/1 -> Data Type Conversion1/1
  Gain/1 -> Bitwise Operator/1
  Data Type Conversion2/1 -> Out1/1

== system AUAV3_AND_SLUGS_SENSOR/Read Barometer BMP180/I2C Initialisation Read EEPROM Calibration data Once (Blocking Function)/Pack12 ==
  Hi : Inport
  Low : Inport  Port=2
  Bitwise Operator : simulink/Logic and Bit Operations/Bitwise Operator  logicop=OR  UseBitMask=off  NumInputPorts=2  BitMask=bin2dec('11011001')  BitMaskRealWorld=Stored Integer
  Data Type Conversion1 : DataTypeConversion  OutDataTypeStr=uint16  ConvertRealWorld=Stored Integer (SI)
  Data Type Conversion2 : DataTypeConversion  OutDataTypeStr=uint16  ConvertRealWorld=Stored Integer (SI)
  Data Type Conversion3 : DataTypeConversion  OutDataTypeStr=uint16  ConvertRealWorld=Stored Integer (SI)
  Gain : Gain  Gain=2^8  OutDataTypeStr=Inherit: Same as input
  Out1 : Outport
  wires:
  Data Type Conversion2/1 -> Out1/1
  Gain/1 -> Bitwise Operator/1
  Hi/1 -> Data Type Conversion1/1
  Bitwise Operator/1 -> Data Type Conversion2/1
  Data Type Conversion1/1 -> Gain/1
  Low/1 -> Data Type Conversion3/1
  Data Type Conversion3/1 -> Bitwise Operator/2

== system AUAV3_AND_SLUGS_SENSOR/Read Barometer BMP180/I2C Initialisation Read EEPROM Calibration data Once (Blocking Function)/Pack2 ==
  Hi : Inport
  Low : Inport  Port=2
  Bitwise Operator : simulink/Logic and Bit Operations/Bitwise Operator  logicop=OR  UseBitMask=off  NumInputPorts=2  BitMask=bin2dec('11011001')  BitMaskRealWorld=Stored Integer
  Data Type Conversion1 : DataTypeConversion  OutDataTypeStr=uint16  ConvertRealWorld=Stored Integer (SI)
  Data Type Conversion2 : DataTypeConversion  OutDataTypeStr=uint16  ConvertRealWorld=Stored Integer (SI)
  Data Type Conversion3 : DataTypeConversion  OutDataTypeStr=uint16  ConvertRealWorld=Stored Integer (SI)
  Gain : Gain  Gain=2^8  OutDataTypeStr=Inherit: Same as input
  Out1 : Outport
  wires:
  Data Type Conversion2/1 -> Out1/1
  Gain/1 -> Bitwise Operator/1
  Hi/1 -> Data Type Conversion1/1
  Bitwise Operator/1 -> Data Type Conversion2/1
  Data Type Conversion1/1 -> Gain/1
  Low/1 -> Data Type Conversion3/1
  Data Type Conversion3/1 -> Bitwise Operator/2

== system AUAV3_AND_SLUGS_SENSOR/Read Barometer BMP180/I2C Initialisation Read EEPROM Calibration data Once (Blocking Function)/Pack3 ==
  Hi : Inport
  Low : Inport  Port=2
  Bitwise Operator : simulink/Logic and Bit Operations/Bitwise Operator  logicop=OR  UseBitMask=off  NumInputPorts=2  BitMask=bin2dec('11011001')  BitMaskRealWorld=Stored Integer
  Data Type Conversion1 : DataTypeConversion  OutDataTypeStr=uint16  ConvertRealWorld=Stored Integer (SI)
  Data Type Conversion2 : DataTypeConversion  OutDataTypeStr=uint16  ConvertRealWorld=Stored Integer (SI)
  Data Type Conversion3 : DataTypeConversion  OutDataTypeStr=uint16  ConvertRealWorld=Stored Integer (SI)
  Gain : Gain  Gain=2^8  OutDataTypeStr=Inherit: Same as input
  Out1 : Outport
  wires:
  Data Type Conversion3/1 -> Bitwise Operator/2
  Low/1 -> Data Type Conversion3/1
  Data Type Conversion1/1 -> Gain/1
  Bitwise Operator/1 -> Data Type Conversion2/1
  Hi/1 -> Data Type Conversion1/1
  Gain/1 -> Bitwise Operator/1
  Data Type Conversion2/1 -> Out1/1

== system AUAV3_AND_SLUGS_SENSOR/Read Barometer BMP180/I2C Initialisation Read EEPROM Calibration data Once (Blocking Function)/Pack4 ==
  Hi : Inport
  Low : Inport  Port=2
  Bitwise Operator : simulink/Logic and Bit Operations/Bitwise Operator  logicop=OR  UseBitMask=off  NumInputPorts=2  BitMask=bin2dec('11011001')  BitMaskRealWorld=Stored Integer
  Data Type Conversion1 : DataTypeConversion  OutDataTypeStr=uint16  ConvertRealWorld=Stored Integer (SI)
  Data Type Conversion2 : DataTypeConversion  OutDataTypeStr=uint16  ConvertRealWorld=Stored Integer (SI)
  Data Type Conversion3 : DataTypeConversion  OutDataTypeStr=uint16  ConvertRealWorld=Stored Integer (SI)
  Gain : Gain  Gain=2^8  OutDataTypeStr=Inherit: Same as input
  Out1 : Outport
  wires:
  Data Type Conversion3/1 -> Bitwise Operator/2
  Low/1 -> Data Type Conversion3/1
  Data Type Conversion1/1 -> Gain/1
  Bitwise Operator/1 -> Data Type Conversion2/1
  Hi/1 -> Data Type Conversion1/1
  Gain/1 -> Bitwise Operator/1
  Data Type Conversion2/1 -> Out1/1

== system AUAV3_AND_SLUGS_SENSOR/Read Barometer BMP180/I2C Initialisation Read EEPROM Calibration data Once (Blocking Function)/Pack5 ==
  Hi : Inport
  Low : Inport  Port=2
  Bitwise Operator : simulink/Logic and Bit Operations/Bitwise Operator  logicop=OR  UseBitMask=off  NumInputPorts=2  BitMask=bin2dec('11011001')  BitMaskRealWorld=Stored Integer
  Data Type Conversion1 : DataTypeConversion  OutDataTypeStr=uint16  ConvertRealWorld=Stored Integer (SI)
  Data Type Conversion2 : DataTypeConversion  OutDataTypeStr=uint16  ConvertRealWorld=Stored Integer (SI)
  Data Type Conversion3 : DataTypeConversion  OutDataTypeStr=uint16  ConvertRealWorld=Stored Integer (SI)
  Gain : Gain  Gain=2^8  OutDataTypeStr=Inherit: Same as input
  Out1 : Outport
  wires:
  Data Type Conversion2/1 -> Out1/1
  Gain/1 -> Bitwise Operator/1
  Hi/1 -> Data Type Conversion1/1
  Bitwise Operator/1 -> Data Type Conversion2/1
  Data Type Conversion1/1 -> Gain/1
  Low/1 -> Data Type Conversion3/1
  Data Type Conversion3/1 -> Bitwise Operator/2

== system AUAV3_AND_SLUGS_SENSOR/Read Barometer BMP180/I2C Initialisation Read EEPROM Calibration data Once (Blocking Function)/Pack6 ==
  Hi : Inport
  Low : Inport  Port=2
  Bitwise Operator : simulink/Logic and Bit Operations/Bitwise Operator  logicop=OR  UseBitMask=off  NumInputPorts=2  BitMask=bin2dec('11011001')  BitMaskRealWorld=Stored Integer
  Data Type Conversion1 : DataTypeConversion  OutDataTypeStr=uint16  ConvertRealWorld=Stored Integer (SI)
  Data Type Conversion2 : DataTypeConversion  OutDataTypeStr=uint16  ConvertRealWorld=Stored Integer (SI)
  Data Type Conversion3 : DataTypeConversion  OutDataTypeStr=uint16  ConvertRealWorld=Stored Integer (SI)
  Gain : Gain  Gain=2^8  OutDataTypeStr=Inherit: Same as input
  Out1 : Outport
  wires:
  Data Type Conversion3/1 -> Bitwise Operator/2
  Low/1 -> Data Type Conversion3/1
  Data Type Conversion1/1 -> Gain/1
  Bitwise Operator/1 -> Data Type Conversion2/1
  Hi/1 -> Data Type Conversion1/1
  Gain/1 -> Bitwise Operator/1
  Data Type Conversion2/1 -> Out1/1

== system AUAV3_AND_SLUGS_SENSOR/Read Barometer BMP180/I2C Initialisation Read EEPROM Calibration data Once (Blocking Function)/Pack7 ==
  Hi : Inport
  Low : Inport  Port=2
  Bitwise Operator : simulink/Logic and Bit Operations/Bitwise Operator  logicop=OR  UseBitMask=off  NumInputPorts=2  BitMask=bin2dec('11011001')  BitMaskRealWorld=Stored Integer
  Data Type Conversion1 : DataTypeConversion  OutDataTypeStr=uint16  ConvertRealWorld=Stored Integer (SI)
  Data Type Conversion2 : DataTypeConversion  OutDataTypeStr=uint16  ConvertRealWorld=Stored Integer (SI)
  Data Type Conversion3 : DataTypeConversion  OutDataTypeStr=uint16  ConvertRealWorld=Stored Integer (SI)
  Gain : Gain  Gain=2^8  OutDataTypeStr=Inherit: Same as input
  Out1 : Outport
  wires:
  Data Type Conversion2/1 -> Out1/1
  Gain/1 -> Bitwise Operator/1
  Hi/1 -> Data Type Conversion1/1
  Bitwise Operator/1 -> Data Type Conversion2/1
  Data Type Conversion1/1 -> Gain/1
  Low/1 -> Data Type Conversion3/1
  Data Type Conversion3/1 -> Bitwise Operator/2

== system AUAV3_AND_SLUGS_SENSOR/Read Barometer BMP180/I2C Initialisation Read EEPROM Calibration data Once (Blocking Function)/Pack8 ==
  Hi : Inport
  Low : Inport  Port=2
  Bitwise Operator : simulink/Logic and Bit Operations/Bitwise Operator  logicop=OR  UseBitMask=off  NumInputPorts=2  BitMask=bin2dec('11011001')  BitMaskRealWorld=Stored Integer
  Data Type Conversion1 : DataTypeConversion  OutDataTypeStr=uint16  ConvertRealWorld=Stored Integer (SI)
  Data Type Conversion2 : DataTypeConversion  OutDataTypeStr=uint16  ConvertRealWorld=Stored Integer (SI)
  Data Type Conversion3 : DataTypeConversion  OutDataTypeStr=uint16  ConvertRealWorld=Stored Integer (SI)
  Gain : Gain  Gain=2^8  OutDataTypeStr=Inherit: Same as input
  Out1 : Outport
  wires:
  Data Type Conversion2/1 -> Out1/1
  Gain/1 -> Bitwise Operator/1
  Hi/1 -> Data Type Conversion1/1
  Bitwise Operator/1 -> Data Type Conversion2/1
  Data Type Conversion1/1 -> Gain/1
  Low/1 -> Data Type Conversion3/1
  Data Type Conversion3/1 -> Bitwise Operator/2

== system AUAV3_AND_SLUGS_SENSOR/Read Barometer BMP180/I2C Initialisation Read EEPROM Calibration data Once (Blocking Function)/Pack9 ==
  Hi : Inport
  Low : Inport  Port=2
  Bitwise Operator : simulink/Logic and Bit Operations/Bitwise Operator  logicop=OR  UseBitMask=off  NumInputPorts=2  BitMask=bin2dec('11011001')  BitMaskRealWorld=Stored Integer
  Data Type Conversion1 : DataTypeConversion  OutDataTypeStr=uint16  ConvertRealWorld=Stored Integer (SI)
  Data Type Conversion2 : DataTypeConversion  OutDataTypeStr=uint16  ConvertRealWorld=Stored Integer (SI)
  Data Type Conversion3 : DataTypeConversion  OutDataTypeStr=uint16  ConvertRealWorld=Stored Integer (SI)
  Gain : Gain  Gain=2^8  OutDataTypeStr=Inherit: Same as input
  Out1 : Outport
  wires:
  Data Type Conversion3/1 -> Bitwise Operator/2
  Low/1 -> Data Type Conversion3/1
  Data Type Conversion1/1 -> Gain/1
  Bitwise Operator/1 -> Data Type Conversion2/1
  Hi/1 -> Data Type Conversion1/1
  Gain/1 -> Bitwise Operator/1
  Data Type Conversion2/1 -> Out1/1

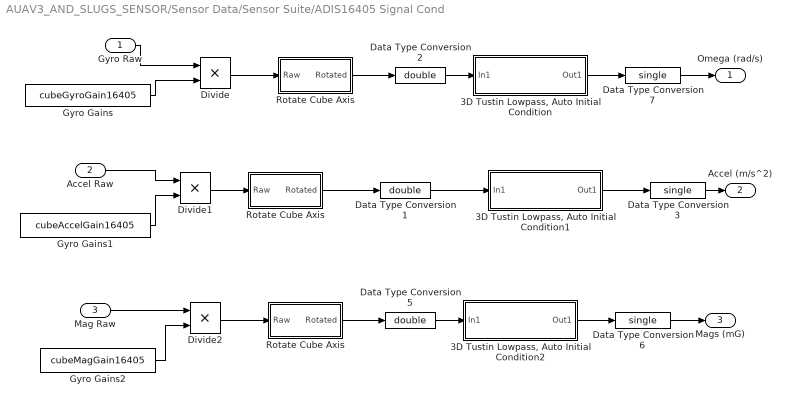
== system AUAV3_AND_SLUGS_SENSOR/Sensor Data/Sensor Suite/ADIS16405 Signal Cond  ==
  Gyro Raw : Inport
  Accel Raw : Inport  Port=2
  Mag Raw : Inport  Port=3
  "3D Tustin Lowpass, Auto Initial Condition" : Subsystem  mask(Tustin1stOrderLowpassAutoInitialCondition){f=mainSensorCutoff, T=T}
      mask prompts: f "Lowpass Frequency"; T "Sample Time"
      mask help: Takes a 3db rolloff frequency (in Hz, NOT radians/s) and a sample time. Performs a symbolic Tustin conversion and implements in a discrete filter. The initial output of the filter is set by the first sample.
      mask Help: Enter the desired 3db rolloff frequency in Hz and the sample time. Initial conditions are sampled automatically.
      mask Display: fprintf('%.2f Hz lowpass (3D)',f)
  "3D Tustin Lowpass, Auto Initial Condition1" : Subsystem  mask(Tustin1stOrderLowpassAutoInitialCondition){f=mainSensorCutoff, T=T}
      mask prompts: f "Lowpass Frequency"; T "Sample Time"
      mask help: Takes a 3db rolloff frequency (in Hz, NOT radians/s) and a sample time. Performs a symbolic Tustin conversion and implements in a discrete filter. The initial output of the filter is set by the first sample.
      mask Help: Enter the desired 3db rolloff frequency in Hz and the sample time. Initial conditions are sampled automatically.
      mask Display: fprintf('%.2f Hz lowpass (3D)',f)
  "3D Tustin Lowpass, Auto Initial Condition2" : Subsystem  mask(Tustin1stOrderLowpassAutoInitialCondition){f=mainSensorCutoff, T=T}
      mask prompts: f "Lowpass Frequency"; T "Sample Time"
      mask help: Takes a 3db rolloff frequency (in Hz, NOT radians/s) and a sample time. Performs a symbolic Tustin conversion and implements in a discrete filter. The initial output of the filter is set by the first sample.
      mask Help: Enter the desired 3db rolloff frequency in Hz and the sample time. Initial conditions are sampled automatically.
      mask Display: fprintf('%.2f Hz lowpass (3D)',f)
  Data Type Conversion1 : DataTypeConversion  OutDataTypeStr=double
  Data Type Conversion2 : DataTypeConversion  OutDataTypeStr=double
  Data Type Conversion3 : DataTypeConversion  OutDataTypeStr=single
  Data Type Conversion5 : DataTypeConversion  OutDataTypeStr=double
  Data Type Conversion6 : DataTypeConversion  OutDataTypeStr=single
  Data Type Conversion7 : DataTypeConversion  OutDataTypeStr=single
  Divide : Product  OutDataTypeStr=single
  Divide1 : Product  OutDataTypeStr=single
  Divide2 : Product  OutDataTypeStr=single
  Gyro Gains : Constant  Value=cubeGyroGain16405  OutDataTypeStr=single
  Gyro Gains1 : Constant  Value=cubeAccelGain16405  OutDataTypeStr=single
  Gyro Gains2 : Constant  Value=cubeMagGain16405  OutDataTypeStr=single
  Rotate Cube Axis : Subsystem
  "Rotate Cube Axis " : Subsystem
  "Rotate Cube Axis  " : Subsystem
  Omega (rad/s) : Outport
  Accel (m/s^2) : Outport  Port=2
  Mags (mG) : Outport  Port=3
  wires:
  Gyro Gains/1 -> Divide/2
  Divide/1 -> Rotate Cube Axis/1(Raw)
  Divide1/1 -> "Rotate Cube Axis "/1(Raw)
  "Rotate Cube Axis "/1(Rotated) -> Data Type Conversion1/1
  Gyro Gains1/1 -> Divide1/2
  Gyro Raw/1 -> Divide/1
  Data Type Conversion2/1 -> "3D Tustin Lowpass, Auto Initial Condition"/1(In1)
  "3D Tustin Lowpass, Auto Initial Condition"/1(Out1) -> Data Type Conversion7/1
  Data Type Conversion7/1 -> Omega (rad/s)/1
  Rotate Cube Axis/1(Rotated) -> Data Type Conversion2/1
  Data Type Conversion1/1 -> "3D Tustin Lowpass, Auto Initial Condition1"/1(In1)
  "3D Tustin Lowpass, Auto Initial Condition1"/1(Out1) -> Data Type Conversion3/1
  Data Type Conversion3/1 -> Accel (m/s^2)/1
  Accel Raw/1 -> Divide1/1
  Divide2/1 -> "Rotate Cube Axis  "/1(Raw)
  Data Type Conversion5/1 -> "3D Tustin Lowpass, Auto Initial Condition2"/1(In1)
  "3D Tustin Lowpass, Auto Initial Condition2"/1(Out1) -> Data Type Conversion6/1
  Data Type Conversion6/1 -> Mags (mG)/1
  "Rotate Cube Axis  "/1(Rotated) -> Data Type Conversion5/1
  Mag Raw/1 -> Divide2/1
  Gyro Gains2/1 -> Divide2/2

== system AUAV3_AND_SLUGS_SENSOR/Sensor Data/Sensor Suite/Compute CPU Load ==
  Calculus Time Step1 : MCHP_Blockset/Profiling/MCU Load  MCULoadPin=Dynamic Options  MCULoadPin_TXT=None  MCULoadMeasure=on  TIMER_Resolution=Dynamic Options  TIMER_Resolution_TXT="Resol: 0.9143(us)  -  Max: 59.9(ms)"  MCHP_TIMER_REQUEST={MCU_Load}{MCU_Load}21:5:0:0:[]:4194304;  MCHP_TIMER_RESULT=[3 65535 ]  MCHP_MASTERLINK=|  MCHP_COMPILED_INFO="CompiledSampleTime= [0.01   0 ];CompiledInportDataTypes=[ ];CompiledInportDataWidth=[];"  Info="Timer 3:  Resol: 914.2857143(ns)  -  Max: 59.9186(ms)"  SampleTime=.01
      | AUAV3_AND_SLUGS_SENSOR/Microchip Master
      | AUAV V3 Board
      | Busy Flag on D2 (RA6)
  Calculus Time Step2 : MCHP_Blockset/Profiling/MCU Overload  MCUOverloadBlockOutput=on  MCUOverLoadPin=Dynamic Options  MCUOverLoadPin_TXT=None  MCHP_MASTERLINK=|  SampleTime=.01
      | AUAV3_AND_SLUGS_SENSOR/Microchip Master
      | AUAV V3 Board
      | Busy Flag on D2 (RA6)
  Data Type Conversion1 : DataTypeConversion  OutDataTypeStr=single
  Data Type Conversion12 : DataTypeConversion  OutDataTypeStr=uint8
  Data Type Conversion2 : DataTypeConversion  OutDataTypeStr=single
  Divide : Product  Inputs=*/  OutDataTypeStr=double
  Gain : Gain  Gain=100
  Rounding Function : Rounding
  Load (%) : Outport
  wires:
  Calculus Time Step1/1 -> Data Type Conversion2/1
  Calculus Time Step2/1 -> Data Type Conversion1/1
  Divide/1 -> Gain/1
  Rounding Function/1 -> Data Type Conversion12/1
  Data Type Conversion1/1 -> Divide/2
  Data Type Conversion2/1 -> Divide/1
  Data Type Conversion12/1 -> Load (%)/1
  Gain/1 -> Rounding Function/1
